simulink library "BrickPi"  (R2018b)
settings: Solver=VariableStepAuto  StartTime=0.0  StopTime=10.0  RelTol=1e-3
libraries: raspberrypilib x50, hdlsllib x27, xpcutilitieslib x18, $bdroot x1
(part 1 of 4)
settings Model: Creator=Isshu  LastModifiedBy=Isshu

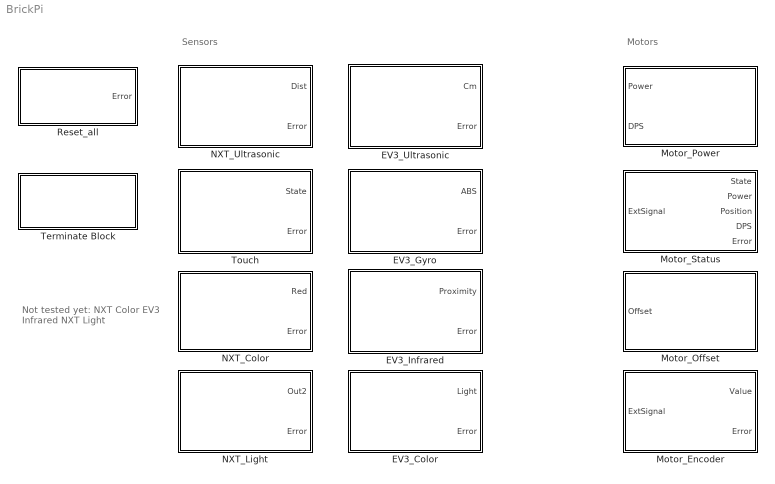
== system BrickPi ==
  note: Not tested yet:
      |
      | NXT Color
      | EV3 Infrared
      | NXT Light
  note: Sensors
  note: Motors
  EV3_Color : Subsystem  mask{SensorPort=1, SensorType=SENSOR_TYPE_EV3_COLOR_AMBIENT}
      mask prompts: SensorPort "Sensor Port"; SensorType "Sensor Type"
      mask init:
      | switch SensorType
      |     case 1, 2
      |         replace_block([gcb, '/Light'],'Terminator','Outport','noprompt')
      |         replace_block([gcb, '/Color_val'],'Outport','Terminator','noprompt')
      |         replace_block([gcb, '/Raw_red'],'Outport','Terminator','noprompt')
      |         replace_block([gcb, '/Red'],'Outport','Terminator','noprompt')
      |         replace_block([gcb, '/Green'],'Outport','Terminator','noprompt')
      |         replace_block([gcb, '/Blue'],'Outport','Terminator','noprompt')
      |         
      |         set_param([gcb, '/Light'],'Port','1')
      |         set_param([gcb, '/Error'],'Port','2')
      |     case 3
      |         replace_block([gcb, '/Light'],'Outport','Terminator','noprompt')
      |         replace_block([gcb, '/Color_val'],'Terminator','Outport','noprompt')
      |         replace_block([gcb, '/Raw_red'],'Outport','Terminator','noprompt')
      |         replace_block([gcb, '/Red'],'Outport','Terminator','noprompt')
      |         replace_block([gcb, '/Green'],'Outport','Terminator','noprompt')
      |         replace_block([gcb, '/Blue'],'Outport','Terminator','noprompt')
      |         
      |         set_param([gcb, '/Color_val'],'Port','1')
      |         set_param([gcb, '/Error'],'Port','2')
      |     case 4
      |         replace_block([gcb, '/Light'],'Outport','Terminator','noprompt')
      |         replace_block([gcb, '/Color_val'],'Outport','Terminator','noprompt')
      |         replace_block([gcb, '/Raw_red'],'Terminator','Outport','noprompt')
      |         replace_block([gcb, '/Red'],'Outport','Terminator','noprompt')
      |         replace_block([gcb, '/Green'],'Outport','Terminator','noprompt')
      |         replace_block([gcb, '/Blue'],'Outport','Terminator','noprompt')
      |         
      |         set_param([gcb, '/Raw_red'],'Port','1')
      |         set_param([gcb, '/Error'],'Port','2')
      |     case 5
      |         replace_block([gcb, '/Light'],'Outport','Terminator','noprompt')
      |         replace_block([gcb, '/Color_val'],'Outport','Terminator','noprompt')
      |         replace_block([gcb, '/Raw_red'],'Outport','Terminator','noprompt')
      |         replace_block([gcb, '/Red'],'Terminator','Outport','noprompt')
      |         replace_block([gcb, '/Green'],'Terminator','Outport','noprompt')
      |         replace_block([gcb, '/Blue'],'Terminator','Outport','noprompt')
      |         
      |         set_param([gcb, '/Red'],'Port','1')
      |         set_param([gcb, '/Green'],'Port','2')
      |         set_param([gcb, '/Blue'],'Port','3')
      |         set_param([gcb, '/Error'],'Port','4')
      | end
      mask TypeOptions SensorPort: 1 | 2 | 3 | 4
      mask TypeOptions SensorType: SENSOR_TYPE_EV3_COLOR_REFLECTED | SENSOR_TYPE_EV3_COLOR_AMBIENT | SENSOR_TYPE_EV3_COLOR_COLOR | SENSOR_TYPE_EV3_COLOR_RAW_REFLECTED | SENSOR_TYPE_EV3_COLOR_COLOR_COMPONENTS
      mask DialogControl DescGroupVar Prompt: EV3 Color Sensor
      mask DialogControl DescTextVar Prompt: <p>         <u>         REFLECTED/ AMBIENT:         </u> <br>         Returns 8 bit integer value for relected light/ light.     </p>     <p>         <u>         COLOR:         </u> <br>         Returns 8 bit integer corresponding to following colors:     </p>         <ul>             <li>0 = No Color</li>             <li>1 = Black</li>             <li>2 = Blue</li>             <li>3 = Green</li>             <li>4 = Yellow</li>             <li>5 = Red</li>             <li>6 = White</li>             <li>7 = Brown</li>         </ul>     <p>         <u>         RAW_REFLECTED:         </u> <br>         Returns 16 bit integer value for measured light.     </p>     <p>         <u>         COLOR_COMPONENTS:         </u> <br>         Returns three 16 bit integer values for red, green and blue and measured light.     </p>
      mask Display:
      | msg = 'EV3 Color\nSensor';
      | switch SensorType
      |     case 1
      |         port_label('output',1,'Light');
      |         port_label('output',2,'Error');
      |     case 2
      |         port_label('output',1,'Light');
      |         port_label('output',2,'Error');
      |     case 3
      |         port_label('output',1,'Color_val');
      |         port_label('output',2,'Error');
      |     case 4
      |         port_label('output',1,'Raw_red');
      |         port_label('output',2,'Error');
      |     case 5
      |         port_label('output',1,'Red');
      |         port_label('output',2,'Green');
      |         port_label('output',3,'Blue');
      |         port_label('output',4,'Error');
      | end
      | 
      | switch SensorPort
      |     case 1
      |         msg = [msg, '\n\nPORT 1'];
      |     case 2
      |         msg = [msg, '\n\nPORT 2'];
      |     case 3
      |         msg = [msg, '\n\nPORT 3'];
      |     case 4
      |         msg = [msg, '\n\nPORT 4'];
      | end
      | 
      | disp(msg);
  EV3_Gyro : Subsystem  mask{SensorPort=1, SensorType=SENSOR_TYPE_EV3_GYRO_ABS}
      mask prompts: SensorPort "Sensor Port"; SensorType "Sensor Type"
      mask init:
      | switch SensorType
      |     case 1
      |         replace_block([gcb, '/ABS'],'Terminator','Outport','noprompt')
      |         replace_block([gcb, '/DPS'],'Outport','Terminator','noprompt')
      |         set_param([gcb, '/ABS'],'Port','1')
      |         set_param([gcb, '/Error'],'Port','2')
      |     case 2
      |         replace_block([gcb, '/ABS'],'Outport','Terminator','noprompt')
      |         replace_block([gcb, '/DPS'],'Terminator','Outport','noprompt')
      |         set_param([gcb, '/DPS'],'Port','1')
      |         set_param([gcb, '/Error'],'Port','2')
      |     case 3
      |         replace_block([gcb, '/ABS'],'Terminator','Outport','noprompt')
      |         replace_block([gcb, '/DPS'],'Terminator','Outport','noprompt')
      |         set_param([gcb, '/ABS'],'Port','1')
      |         set_param([gcb, '/DPS'],'Port','2')
      |         set_param([gcb, '/Error'],'Port','3')
      | end
      mask TypeOptions SensorPort: 1 | 2 | 3 | 4
      mask TypeOptions SensorType: SENSOR_TYPE_EV3_GYRO_ABS | SENSOR_TYPE_EV3_GYRO_DPS | SENSOR_TYPE_EV3_GYRO_ABS_DPS
      mask DialogControl DescGroupVar Prompt: EV3 Gyro Sensor
      mask DialogControl DescTextVar Prompt: <p>         <u>         ABS:         </u> <br>         Returns 16 bit integer value for measured gyro angle in deg.     </p>     <p>         <u>         DPS:         </u> <br>         Returns 16 bit integer value for measured gyro angle velocity in deg/s.     </p>     <p>         <u>         ABD_DPS:         </u> <br>         Returns two 16 bit integer values, one for gyro angle and one for gyro angle velocity.     </p>
      mask Display:
      | msg = 'EV3 Gyro\nSensor';
      | switch SensorType
      |     case 1
      |         port_label('output',1,'ABS');
      |         port_label('output',2,'Error');
      |     case 2
      |         port_label('output',1,'DPS');
      |         port_label('output',2,'Error');
      |     case 3
      |         port_label('output',1,'ABS');
      |         port_label('output',2,'DPS');
      |         port_label('output',3,'Error');
      | end
      | 
      | switch SensorPort
      |     case 1
      |         msg = [msg, '\n\nPORT 1'];
      |     case 2
      |         msg = [msg, '\n\nPORT 2'];
      |     case 3
      |         msg = [msg, '\n\nPORT 3'];
      |     case 4
      |         msg = [msg, '\n\nPORT 4'];
      | end
      | 
      | disp(msg);
  EV3_Infrared : Subsystem  mask{SensorPort=1, SensorType=SENSOR_TYPE_EV3_INFRARED_PROXIMITY}
      mask prompts: SensorPort "Sensor Port"; SensorType "Sensor Type"
      mask init:
      | switch SensorType
      |     case 1
      |         replace_block([gcb, '/Proximity'],'Terminator','Outport','noprompt')
      |         replace_block([gcb, '/Heading'],'Outport','Terminator','noprompt')
      |         replace_block([gcb, '/Distance'],'Outport','Terminator','noprompt')
      |         replace_block([gcb, '/Remote'],'Outport','Terminator','noprompt')
      |         set_param([gcb, '/Proximity'],'Port','1')
      |         set_param([gcb, '/Error'],'Port','2')
      |     case 2
      |         replace_block([gcb, '/Proximity'],'Outport','Terminator','noprompt')
      |         replace_block([gcb, '/Heading'],'Terminator','Outport','noprompt')
      |         replace_block([gcb, '/Distance'],'Terminator','Outport','noprompt')
      |         replace_block([gcb, '/Remote'],'Outport','Terminator','noprompt')
      |         set_param([gcb, '/Heading'],'Port','1')
      |         set_param([gcb, '/Distance'],'Port','2')
      |         set_param([gcb, '/Error'],'Port','3')
      |     case 3
      |         replace_block([gcb, '/Proximity'],'Outport','Terminator','noprompt')
      |         replace_block([gcb, '/Heading'],'Outport','Terminator','noprompt')
      |         replace_block([gcb, '/Distance'],'Outport','Terminator','noprompt')
      |         replace_block([gcb, '/Remote'],'Terminator','Outport','noprompt')
      |         set_param([gcb, '/Remote'],'Port','1')
      |         set_param([gcb, '/Error'],'Port','2')
      | end
      mask TypeOptions SensorPort: 1 | 2 | 3 | 4
      mask TypeOptions SensorType: SENSOR_TYPE_EV3_INFRARED_PROXIMITY | SENSOR_TYPE_EV3_INFRARED_SEEK | SENSOR_TYPE_EV3_INFRARED_REMOTE
      mask Display:
      | msg = 'EV3 Infrared\nSensor';
      | switch SensorType
      |     case 1
      |         port_label('output',1,'Proximity');
      |         port_label('output',2,'Error');
      |     case 2
      |         port_label('output',1,'Heading');
      |         port_label('output',2,'Distance');
      |         port_label('output',3,'Error');
      |     case 3
      |         port_label('output',1,'Remote');
      |         port_label('output',2,'Error');
      | end
      | 
      | switch SensorPort
      |     case 1
      |         msg = [msg, '\n\nPORT 1'];
      |     case 2
      |         msg = [msg, '\n\nPORT 2'];
      |     case 3
      |         msg = [msg, '\n\nPORT 3'];
      |     case 4
      |         msg = [msg, '\n\nPORT 4'];
      | end
      | 
      | disp(msg);
  EV3_Ultrasonic : Subsystem  mask{SensorPort=1, SensorType=SENSOR_TYPE_EV3_ULTRASONIC_CM}
      mask prompts: SensorPort "Sensor Port"; SensorType "Sensor Type"
      mask init:
      | switch SensorType
      |     case 1
      |         replace_block([gcb, '/Cm'],'Terminator','Outport','noprompt')
      |         replace_block([gcb, '/Inches'],'Outport','Terminator','noprompt')
      |         replace_block([gcb, '/Pres'],'Outport','Terminator','noprompt')
      |         set_param([gcb, '/Cm'],'Port','1')
      |         set_param([gcb, '/Error'],'Port','2')
      |     case 2
      |         replace_block([gcb, '/Cm'],'Outport','Terminator','noprompt')
      |         replace_block([gcb, '/Inches'],'Terminator','Outport','noprompt')
      |         replace_block([gcb, '/Pres'],'Outport','Terminator','noprompt')
      |         set_param([gcb, '/Inches'],'Port','1')
      |         set_param([gcb, '/Error'],'Port','2')
      |     case 3
      |         replace_block([gcb, '/Cm'],'Outport','Terminator','noprompt')
      |         replace_block([gcb, '/Inches'],'Outport','Terminator','noprompt')
      |         replace_block([gcb, '/Pres'],'Terminator','Outport','noprompt')
      |         set_param([gcb, '/Pres'],'Port','1')
      |         set_param([gcb, '/Error'],'Port','2')
      | end
      mask TypeOptions SensorPort: 1 | 2 | 3 | 4
      mask TypeOptions SensorType: SENSOR_TYPE_EV3_ULTRASONIC_CM | SENSOR_TYPE_ EV3_ULTRASONIC_INCHES | SENSOR_TYPE_EV3_ULTRASONIC_LISTEN
      mask DialogControl DescGroupVar Prompt: EV3 Ultrasonic Sensor
      mask DialogControl DescTextVar Prompt: <p>         <u>         CM/ INCHES:         </u> <br>         Returns 16 bit float value for measured distance in cm/ inches.     </p>     <p>         <u>         LISTEN:         </u> <br>         Returns boolean value for presence.     </p>
      mask Display:
      | msg = 'EV3 Ultrasonic\nSensor';
      | 
      | switch SensorType
      |     case 1
      |         port_label('output',1,'Cm');
      |         port_label('output',2,'Error');
      |     case 2
      |         port_label('output',1,'Inches');
      |         port_label('output',2,'Error');
      |     case 3
      |         port_label('output',1,'Pres');
      |         port_label('output',2,'Error');
      | end
      | 
      | switch SensorPort
      |     case 1
      |         msg = [msg, '\n\nPORT 1'];
      |     case 2
      |         msg = [msg, '\n\nPORT 2'];
      |     case 3
      |         msg = [msg, '\n\nPORT 3'];
      |     case 4
      |         msg = [msg, '\n\nPORT 4'];
      | end
      | 
      | disp(msg);
  Motor_Encoder : Subsystem  mask{MotorPort=A, ResetMode=Reset on external signal}
      mask prompts: MotorPort "Motor Port"; ResetMode "Encoder Reset"
      mask init:
      | switch ResetMode
      |     case 1
      |         replace_block([gcb,'/ExtSignal'],'Ground','Inport','noprompt')
      |     otherwise
      |         replace_block([gcb,'/ExtSignal'],'Inport','Ground','noprompt')
      | end
      mask TypeOptions MotorPort: A | B | C | D
      mask TypeOptions ResetMode: Reset on external signal | Never reset
      mask DialogControl DescGroupVar Prompt: Get Motor Encoder
      mask DialogControl DescTextVar Prompt: <p>         Optionally one can decide whether the motor encoder is reset while program is running. For example use "Pulse generator" to reset encoder every fixed timestep.     </p>          <p>         Returns int32 value for motor encoder value.     </p>
      mask Display:
      | msg = 'Get Motor\nEncoder';
      | port_label('output',1,'Value');
      | port_label('output',2,'Error');
      | 
      | if ResetMode==1
      |         port_label('input',1,'Reset');
      | end
      | 
      | switch MotorPort
      |     case 1
      |         msg = [msg, '\n\nPORT A'];
      |     case 2
      |         msg = [msg, '\n\nPORT B'];
      |     case 3
      |         msg = [msg, '\n\nPORT C'];
      |     case 4
      |         msg = [msg, '\n\nPORT D'];
      | end
      | 
      | disp(msg);
  Motor_Offset : Subsystem  mask{MotorPort=A}
      mask prompts: MotorPort "Motor Port"
      mask TypeOptions MotorPort: A | B | C | D
      mask DialogControl DescGroupVar Prompt: Set Motor Offset
      mask DialogControl DescTextVar Prompt: <p>         Set int32 value for motor encoder offset.     </p>
      mask Display:
      | port_label('input',1,'Offset');
      | msg = 'Set Motor\nOffset';
      | 
      | switch MotorPort
      |     case 1
      |         msg = [msg, '\n\nPORT A'];
      |     case 2
      |         msg = [msg, '\n\nPORT B'];
      |     case 3
      |         msg = [msg, '\n\nPORT C'];
      |     case 4
      |         msg = [msg, '\n\nPORT D'];
      | end
      | 
      | disp(msg);
  Motor_Power : Subsystem  mask{MotorPort=A, choice=Limits, Kp=0, Kd=0, Kp_DPS=0, Kd_DPS=0}
      mask prompts: MotorPort "Motor Port"; choice "Set Motor"; Kp_DPS "Kp for DPS"; Kd_DPS "Kp for DPS"
      mask init:
      | switch choice
      |     case 1
      |         replace_block([gcb, '/Power'],'Ground','Inport','noprompt')
      |         replace_block([gcb, '/Position'],'Inport','Ground','noprompt')
      |         replace_block([gcb, '/DPS'],'Inport','Ground','noprompt')
      |         
      |         set_param([gcb, '/Power'],'Port','1')
      |     case 2
      |         replace_block([gcb, '/Power'],'Inport','Ground','noprompt')
      |         replace_block([gcb, '/Position'],'Ground','Inport','noprompt')
      |         replace_block([gcb, '/DPS'],'Inport','Ground','noprompt')
      |         
      |         set_param([gcb, '/Position'],'Port','1')
      |     case 3
      |         replace_block([gcb, '/Power'],'Inport','Ground','noprompt')
      |         replace_block([gcb, '/Position'],'Inport','Ground','noprompt')
      |         replace_block([gcb, '/DPS'],'Ground','Inport','noprompt')
      |         
      |         set_param([gcb, '/DPS'],'Port','1')
      |     case 4
      |         replace_block([gcb, '/Power'],'Ground','Inport','noprompt')
      |         replace_block([gcb, '/Position'],'Inport','Ground','noprompt')
      |         replace_block([gcb, '/DPS'],'Ground','Inport','noprompt')
      |         
      |         set_param([gcb, '/Power'],'Port','1')
      |         set_param([gcb, '/DPS'],'Port','2')
      | end
      mask TypeOptions MotorPort: A | B | C | D
      mask TypeOptions choice: Power | Position | DPS | Limits
      mask DialogControl DescGroupVar Prompt: Set Motor Properties
      mask DialogControl DescTextVar Prompt: <p>         <u>POWER</u> <br>         Set 8 bit signed integer value for motor power. -128 stops motor.     </p>     <p>         <u>POSITION</u> <br>         Set 32 bit signed integer value for motor position.     </p>     <p>         <u>DPS</u> <br>         Set 16 bit signed integer value for motor angle velocity.     </p>     <p>         <u>LIMITS</u> <br>         Set 8 bit unsigned integer value for power and 16 bit unsigned integer value for motor angle velocity.     </p> <p>Optionally Kp and Kd values for motor position and dps control can be set. They are set as soon as the values are changed. If every K value is set to zero position control won't work anymore. In that case tune Kp for example to 10. Default values are unfortunately not known.</p>
      mask Display:
      | switch choice
      |     case 1
      |         port_label('input',1,'Power');
      |         msg = 'Set Motor\nPower';
      |     case 2
      |         port_label('input',1,'Position');
      |         msg = 'Set Motor\nPosition';
      |     case 3
      |         port_label('input',1,'DPS');
      |         msg = 'Set Motor\nDPS';
      |     case 4
      |         port_label('input',1,'Power');
      |         port_label('input',2,'DPS');
      |         msg = 'Set Motor\nLimits';
      | end
      | 
      | switch MotorPort
      |     case 1
      |         msg = [msg, '\n\nPORT A'];
      |     case 2
      |         msg = [msg, '\n\nPORT B'];
      |     case 3
      |         msg = [msg, '\n\nPORT C'];
      |     case 4
      |         msg = [msg, '\n\nPORT D'];
      | end
      | 
      | disp(msg);
  Motor_Status : Subsystem  mask{MotorPort=A, ResetMode=Reset on external signal}
      mask prompts: MotorPort "Motor Port"; ResetMode "Encoder Reset"
      mask init:
      | switch ResetMode
      |     case 1
      |         replace_block([gcb,'/ExtSignal'],'Ground','Inport','noprompt')
      |     otherwise
      |         replace_block([gcb,'/ExtSignal'],'Inport','Ground','noprompt')
      | end
      mask TypeOptions MotorPort: A | B | C | D
      mask TypeOptions ResetMode: Reset on external signal | Never reset
      mask DialogControl DescGroupVar Prompt: Get Motor Status
      mask DialogControl DescTextVar Prompt: <p>         Returns uint8 integer value for motor state, int8 value for power, int32 value for position and int16 value for motor angle velocity.     </p>          <p>         Optionally one can decide whether the motor encoder is reset while program is running. For example use "Pulse generator" to reset encoder every fixed timestep.     </p>
      mask Display:
      | msg = 'Get Motor\nStatus';
      | port_label('output',1,'State');
      | port_label('output',2,'Power');
      | port_label('output',3,'Position');
      | port_label('output',4,'DPS');
      | port_label('output',5,'Error');
      | 
      | if ResetMode==1
      |         port_label('input',1,'Reset');
      | end
      | 
      | switch MotorPort
      |     case 1
      |         msg = [msg, '\n\nPORT A'];
      |     case 2
      |         msg = [msg, '\n\nPORT B'];
      |     case 3
      |         msg = [msg, '\n\nPORT C'];
      |     case 4
      |         msg = [msg, '\n\nPORT D'];
      | end
      | 
      | disp(msg);
  NXT_Color : Subsystem  mask{SensorPort=1, SensorType=SENSOR_TYPE_NXT_COLOR_RED}
      mask prompts: SensorPort "Sensor Port"; SensorType "Sensor Type"
      mask init:
      | switch SensorType
      |     case 1
      |         replace_block([gcb, '/Red'],'Terminator','Outport','noprompt')
      |         replace_block([gcb, '/Green'],'Outport','Terminator','noprompt')
      |         replace_block([gcb, '/Blue'],'Outport','Terminator','noprompt')
      |         replace_block([gcb, '/Color'],'Outport','Terminator','noprompt')
      |         replace_block([gcb, '/Ambient'],'Outport','Terminator','noprompt')
      |         
      |         set_param([gcb, '/Red'],'Port','1')
      |         set_param([gcb, '/Error'],'Port','2')
      |     case 2
      |         replace_block([gcb, '/Red'],'Outport','Terminator','noprompt')
      |         replace_block([gcb, '/Green'],'Terminator','Outport','noprompt')
      |         replace_block([gcb, '/Blue'],'Outport','Terminator','noprompt')
      |         replace_block([gcb, '/Color'],'Outport','Terminator','noprompt')
      |         replace_block([gcb, '/Ambient'],'Outport','Terminator','noprompt')
      |         
      |         set_param([gcb, '/Green'],'Port','1')
      |         set_param([gcb, '/Error'],'Port','2')
      |     case 3
      |         replace_block([gcb, '/Red'],'Outport','Terminator','noprompt')
      |         replace_block([gcb, '/Green'],'Outport','Terminator','noprompt')
      |         replace_block([gcb, '/Blue'],'Terminator','Outport','noprompt')
      |         replace_block([gcb, '/Color'],'Outport','Terminator','noprompt')
      |         replace_block([gcb, '/Ambient'],'Outport','Terminator','noprompt')
      |         
      |         set_param([gcb, '/Blue'],'Port','1')
      |         set_param([gcb, '/Error'],'Port','2')
      |     case 4
      |         replace_block([gcb, '/Red'],'Terminator','Outport','noprompt')
      |         replace_block([gcb, '/Green'],'Terminator','Outport','noprompt')
      |         replace_block([gcb, '/Blue'],'Terminator','Outport','noprompt')
      |         replace_block([gcb, '/Color'],'Terminator','Outport','noprompt')
      |         replace_block([gcb, '/Ambient'],'Terminator','Outport','noprompt')
      |         
      |         set_param([gcb, '/Red'],'Port','1')
      |         set_param([gcb, '/Green'],'Port','2')
      |         set_param([gcb, '/Blue'],'Port','3')
      |         set_param([gcb, '/Color'],'Port','4')
      |         set_param([gcb, '/Ambient'],'Port','5')
      |         set_param([gcb, '/Error'],'Port','6')
      |     case 5
      |         replace_block([gcb, '/Red'],'Outport','Terminator','noprompt')
      |         replace_block([gcb, '/Green'],'Outport','Terminator','noprompt')
      |         replace_block([gcb, '/Blue'],'Outport','Terminator','noprompt')
      |         replace_block([gcb, '/Color'],'Outport','Terminator','noprompt')
      |         replace_block([gcb, '/Ambient'],'Terminator','Outport','noprompt')
      |         
      |         set_param([gcb, '/Ambient'],'Port','1')
      |         set_param([gcb, '/Error'],'Port','2')
      | end
      mask TypeOptions SensorPort: 1 | 2 | 3 | 4
      mask TypeOptions SensorType: SENSOR_TYPE_NXT_COLOR_RED | SENSOR_TYPE_NXT_COLOR_GREEN | SENSOR_TYPE_NXT_COLOR_BLUE | SENSOR_TYPE_NXT_COLOR_FULL | SENSOR_TYPE_NXT_COLOR_OFF
      mask DialogControl DescGroupVar Prompt: NXT Color Sensor
      mask DialogControl DescTextVar Prompt: <p>         <u>         RED/ GREEN/ BLUE/ OFF:         </u> <br>         Returns 16 bit integer value for red/ green/ blue/ measured light.     </p>     <p>         <u>         FULL:         </u> <br>         Returns one 8 bit value for color corresponding to following colors and four 16 bit integer values for red, green, blue and measured light.     </p>     <ul>             <li>0 = No Color</li>             <li>1 = Black</li>             <li>2 = Blue</li>             <li>3 = Green</li>             <li>4 = Yellow</li>             <li>5 = Red</li>             <li>6 = White</li>             <li>7 = Brown</li>     </ul>
      mask Display:
      | msg = 'NXT Color\nSensor';
      | switch SensorType
      |     case 1
      |         port_label('output',1,'Red');
      |         port_label('output',2,'Error');
      |     case 2
      |         port_label('output',1,'Green');
      |         port_label('output',2,'Error');
      |     case 3
      |         port_label('output',1,'Blue');
      |         port_label('output',2,'Error');
      |     case 4
      |         port_label('output',1,'Red');
      |         port_label('output',2,'Green');
      |         port_label('output',3,'Blue');
      |         port_label('output',4,'Color');
      |         port_label('output',5,'Ambient');
      |         port_label('output',6,'Error');
      |     case 5
      |         port_label('output',1,'Amb');
      |         port_label('output',2,'Error');
      | end
      | 
      | switch SensorPort
      |     case 1
      |         msg = [msg, '\n\nPORT 1'];
      |     case 2
      |         msg = [msg, '\n\nPORT 2'];
      |     case 3
      |         msg = [msg, '\n\nPORT 3'];
      |     case 4
      |         msg = [msg, '\n\nPORT 4'];
      | end
      | 
      | disp(msg);
  NXT_Light : Subsystem  mask{SensorPort=1, SensorType=SENSOR_TYPE_NXT_LIGHT_ON}
      mask prompts: SensorPort "Sensor Port"; SensorType "Sensor Type"
      mask TypeOptions SensorPort: 1 | 2 | 3 | 4
      mask TypeOptions SensorType: SENSOR_TYPE_NXT_LIGHT_ON | SENSOR_TYPE_NXT_LIGHT_OFF
      mask DialogControl DescGroupVar Prompt: NXT Light Sensor
      mask DialogControl DescTextVar Prompt: <p>         <u>         ON/ OFF:         </u> <br>         Returns 16 bit integer value for reflected/ measured light.     </p>
      mask Display:
      | msg = 'NXT Light\nSensor';
      | port_label('output',1,'Light');
      | port_label('output',2,'Error');
      | 
      | switch SensorPort
      |     case 1
      |         msg = [msg, '\n\nPORT 1'];
      |     case 2
      |         msg = [msg, '\n\nPORT 2'];
      |     case 3
      |         msg = [msg, '\n\nPORT 3'];
      |     case 4
      |         msg = [msg, '\n\nPORT 4'];
      | end
      | 
      | disp(msg);
  NXT_Ultrasonic : Subsystem  mask{SensorPort=1}
      mask prompts: SensorPort "Sensor Port"
      mask TypeOptions SensorPort: 1 | 2 | 3 | 4
      mask DialogControl DescGroupVar Prompt: NXT Ultrasonic Sensor
      mask DialogControl DescTextVar Prompt: <p>     Returns measured distance in cm as a 8 bit integer value. </p>
      mask Display:
      | msg = 'NXT Ultrasonic\nSensor';
      | port_label('output',1,'Dist');
      | port_label('output',2,'Error');
      | 
      | switch SensorPort
      |     case 1
      |         msg = [msg, '\n\nPORT 1'];
      |     case 2
      |         msg = [msg, '\n\nPORT 2'];
      |     case 3
      |         msg = [msg, '\n\nPORT 3'];
      |     case 4
      |         msg = [msg, '\n\nPORT 4'];
      | end
      | 
      | disp(msg);
  Reset_all : Subsystem
      mask DialogControl DescGroupVar Prompt: Reset
      mask DialogControl DescTextVar Prompt: Sets motor power to -128 (no motion) and resets sensor types assigned to ports
      mask Display: disp('Reset all')
  Terminate Block : Subsystem  TreatAsAtomicUnit=on
  Touch : Subsystem  mask{SensorPort=1, SensorType=SENSOR_TYPE_TOUCH_NXT}
      mask prompts: SensorPort "Sensor Port"; SensorType "Sensor Type"
      mask TypeOptions SensorPort: 1 | 2 | 3 | 4
      mask TypeOptions SensorType: SENSOR_TYPE_TOUCH_NXT | SENSOR_TYPE_TOUCH_EV3
      mask DialogControl DescGroupVar Prompt: NXT/EV3 Touch Sensor
      mask DialogControl DescTextVar Prompt: <p>     Doesn't work if the wrong sensor type (NXT or EV3) is selected. </p> <p>     Returns boolean value for button pushed (1) or not (0). </p>
      mask Display:
      | msg = 'NXT/ EV3 Touch\nSensor';
      | port_label('output',1,'State');
      | port_label('output',2,'Error');
      | 
      | switch SensorPort
      |     case 1
      |         msg = [msg, '\n\nPORT 1'];
      |     case 2
      |         msg = [msg, '\n\nPORT 2'];
      |     case 3
      |         msg = [msg, '\n\nPORT 3'];
      |     case 4
      |         msg = [msg, '\n\nPORT 4'];
      | end
      | 
      | disp(msg);

== system BrickPi/EV3_Color ==
  AND : Logic  AllPortsSameDT=off  OutDataTypeStr=boolean
  Blue : Terminator
  Color_val : Terminator
  Constant : Constant
  Demux : Demux  Outputs=3
  Get_sensor_value : Subsystem
  Green : Terminator
  Memory : Memory
  Mux : Mux  Inputs=2
  NOT : Logic  Operator=NOT  IconShape=distinctive  AllPortsSameDT=off  OutDataTypeStr=boolean
  NOT1 : Logic  Operator=NOT  IconShape=distinctive  AllPortsSameDT=off  OutDataTypeStr=boolean
  Raw_red : Terminator
  Red : Terminator
  SensorPort : Constant  Value=SensorPort  OutDataTypeStr=uint8
  SensorType : Constant  Value=SensorType  OutDataTypeStr=uint8
  Set_sensor_type : Subsystem  Priority=21
  Light : Outport
  Error : Outport  Port=2
  wires:
  SensorType/1 -> Get_sensor_value/2(SensorType), Set_sensor_type/2(SensorType)
  NOT/1 -> Set_sensor_type/Enable
  Mux/1 -> Error/1
  Constant/1 -> Memory/1
  Get_sensor_value/5(Error) -> Mux/2
  Memory/1 -> NOT/1, AND/2
  AND/1 -> Get_sensor_value/Enable
  SensorPort/1 -> Set_sensor_type/1(SensorPort), Get_sensor_value/1(SensorPort)
  Get_sensor_value/1(Light) -> Light/1
  Set_sensor_type/1(Error) -> NOT1/1, Mux/1
  NOT1/1 -> AND/1
  Demux/1 -> Red/1
  Demux/2 -> Green/1
  Demux/3 -> Blue/1
  Get_sensor_value/4(Color) -> Demux/1
  Get_sensor_value/2(Color_val) -> Color_val/1
  Get_sensor_value/3(Raw_red) -> Raw_red/1

== system BrickPi/EV3_Gyro ==
  AND : Logic  AllPortsSameDT=off  OutDataTypeStr=boolean
  Constant : Constant
  DPS : Terminator
  Get_sensor_value : Subsystem
  Memory : Memory
  Mux : Mux  Inputs=2
  NOT : Logic  Operator=NOT  IconShape=distinctive  AllPortsSameDT=off  OutDataTypeStr=boolean
  NOT1 : Logic  Operator=NOT  IconShape=distinctive  AllPortsSameDT=off  OutDataTypeStr=boolean
  SensorPort : Constant  Value=SensorPort  OutDataTypeStr=uint8
  SensorType : Constant  Value=SensorType  OutDataTypeStr=uint8
  Set_sensor_type : Subsystem  Priority=21
  ABS : Outport
  Error : Outport  Port=2
  wires:
  SensorType/1 -> Get_sensor_value/2(SensorType), Set_sensor_type/2(SensorType)
  NOT/1 -> Set_sensor_type/Enable
  Mux/1 -> Error/1
  Constant/1 -> Memory/1
  Get_sensor_value/3(Error) -> Mux/2
  Memory/1 -> NOT/1, AND/2
  AND/1 -> Get_sensor_value/Enable
  SensorPort/1 -> Set_sensor_type/1(SensorPort), Get_sensor_value/1(SensorPort)
  Set_sensor_type/1(Error) -> NOT1/1, Mux/1
  NOT1/1 -> AND/1
  Get_sensor_value/1(ABS) -> ABS/1
  Get_sensor_value/2(DPS) -> DPS/1

== system BrickPi/EV3_Infrared ==
  AND : Logic  AllPortsSameDT=off  OutDataTypeStr=boolean
  Constant : Constant
  Distance : Terminator
  Get_sensor_value : Subsystem
  Heading : Terminator
  Memory : Memory
  Mux : Mux  Inputs=2
  NOT : Logic  Operator=NOT  IconShape=distinctive  AllPortsSameDT=off  OutDataTypeStr=boolean
  NOT1 : Logic  Operator=NOT  IconShape=distinctive  AllPortsSameDT=off  OutDataTypeStr=boolean
  Remote : Terminator
  SensorPort : Constant  Value=SensorPort  OutDataTypeStr=uint8
  SensorType : Constant  Value=SensorType  OutDataTypeStr=uint8
  Set_sensor_type : Subsystem  Priority=21
  Proximity : Outport
  Error : Outport  Port=2
  wires:
  Get_sensor_value/1(Proximity) -> Proximity/1
  Mux/1 -> Error/1
  Set_sensor_type/1(Error) -> Mux/1, NOT1/1
  AND/1 -> Get_sensor_value/Enable
  NOT1/1 -> AND/1
  SensorPort/1 -> Get_sensor_value/1(SensorPort), Set_sensor_type/1(SensorPort)
  Memory/1 -> AND/2, NOT/1
  Constant/1 -> Memory/1
  NOT/1 -> Set_sensor_type/Enable
  SensorType/1 -> Set_sensor_type/2(SensorType), Get_sensor_value/2(SensorType)
  Get_sensor_value/5(Error) -> Mux/2
  Get_sensor_value/4(Remote) -> Remote/1
  Get_sensor_value/3(Distance) -> Distance/1
  Get_sensor_value/2(Heading) -> Heading/1

== system BrickPi/EV3_Ultrasonic ==
  AND : Logic  AllPortsSameDT=off  OutDataTypeStr=boolean
  Constant : Constant
  Get_sensor_value : Subsystem
  Inches : Terminator
  Memory : Memory
  Mux : Mux  Inputs=2
  NOT : Logic  Operator=NOT  IconShape=distinctive  AllPortsSameDT=off  OutDataTypeStr=boolean
  NOT1 : Logic  Operator=NOT  IconShape=distinctive  AllPortsSameDT=off  OutDataTypeStr=boolean
  Pres : Terminator
  SensorPort : Constant  Value=SensorPort  OutDataTypeStr=uint8
  SensorType : Constant  Value=SensorType  OutDataTypeStr=uint8
  Set_sensor_type : Subsystem  Priority=21
  Cm : Outport
  Error : Outport  Port=2
  wires:
  Mux/1 -> Error/1
  Memory/1 -> NOT/1, AND/2
  NOT1/1 -> AND/1
  Get_sensor_value/1(cm) -> Cm/1
  AND/1 -> Get_sensor_value/Enable
  NOT/1 -> Set_sensor_type/Enable
  Get_sensor_value/4(Error) -> Mux/2
  Set_sensor_type/1(Error) -> NOT1/1, Mux/1
  Constant/1 -> Memory/1
  Get_sensor_value/3(pres) -> Pres/1
  SensorPort/1 -> Get_sensor_value/1(SensorPort), Set_sensor_type/1(SensorPort)
  SensorType/1 -> Get_sensor_value/2(SensorType), Set_sensor_type/2(SensorType)
  Get_sensor_value/2(inch) -> Inches/1

== system BrickPi/Motor_Encoder ==
  ExtSignal : Inport
  AND : Logic  IconShape=distinctive  AllPortsSameDT=off  OutDataTypeStr=boolean
  Constant : Constant
  Get Encoder Value : Subsystem
  Memory : Memory
  MotorPort : Constant  Value=MotorPort  OutDataTypeStr=uint8
  NOT : Logic  Operator=NOT  IconShape=distinctive  AllPortsSameDT=off  OutDataTypeStr=boolean
  NOT1 : Logic  Operator=NOT  IconShape=distinctive  AllPortsSameDT=off  OutDataTypeStr=boolean
  Reset Encoder once : Subsystem
  ResetMode : Constant  Value=ResetMode
  Value : Outport
  Error : Outport  Port=2
  wires:
  Get Encoder Value/1(Value) -> Value/1
  Get Encoder Value/2(Error) -> Error/1
  Constant/1 -> Memory/1
  Memory/1 -> NOT1/1, AND/1
  MotorPort/1 -> Get Encoder Value/1(MotorPort), Reset Encoder once/1(MotorPort)
  Reset Encoder once/1(Error) -> NOT/1
  AND/1 -> Get Encoder Value/Enable
  NOT/1 -> AND/2
  ResetMode/1 -> Get Encoder Value/2(ResetMode)
  ExtSignal/1 -> Get Encoder Value/3(ExtSignal)
  NOT1/1 -> Reset Encoder once/Enable

== system BrickPi/Motor_Offset ==
  Offset : Inport  OutDataTypeStr=int32
  If : If  NumInputs=2  IfExpression=u1 ~= u2
  If Action Subsystem : Subsystem  TreatAsAtomicUnit=on
  Memory : Memory
  Terminator : Terminator
  wires:
  If/1 -> If Action Subsystem/Action
  If/2 -> Terminator/1
  Memory/1 -> If/1
  Offset/1 -> If Action Subsystem/1(Offset), If/2, Memory/1

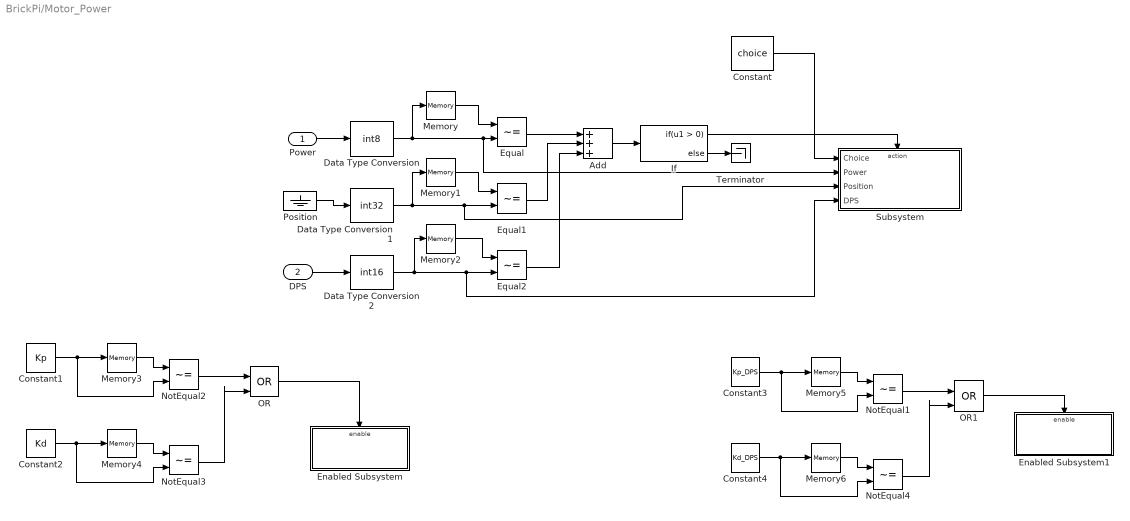
== system BrickPi/Motor_Power ==
  Power : Inport
  DPS : Inport  Port=2
  Add : Sum  Inputs=3
  Constant : Constant  Value=choice
  Constant1 : Constant  Value=Kp
  Constant2 : Constant  Value=Kd
  Constant3 : Constant  Value=Kp_DPS
  Constant4 : Constant  Value=Kd_DPS
  Data Type Conversion : DataTypeConversion  OutDataTypeStr=int8
  Data Type Conversion1 : DataTypeConversion  OutDataTypeStr=int32
  Data Type Conversion2 : DataTypeConversion  OutDataTypeStr=int16
  Enabled Subsystem : Subsystem  TreatAsAtomicUnit=on
  Enabled Subsystem1 : Subsystem  TreatAsAtomicUnit=on
  Equal : RelationalOperator  Operator=~=  RndMeth=Simplest
  Equal1 : RelationalOperator  Operator=~=  RndMeth=Simplest
  Equal2 : RelationalOperator  Operator=~=  RndMeth=Simplest
  If : If
  Memory : Memory  InheritSampleTime=on
  Memory1 : Memory  InheritSampleTime=on
  Memory2 : Memory  InheritSampleTime=on
  Memory{3..6} (4 alike) : Memory
  NotEqual{1..4} (4 alike) : RelationalOperator  Operator=~=  OutDataTypeStr=boolean  RndMeth=Simplest
  OR : Logic  Operator=OR  IconShape=distinctive  AllPortsSameDT=off  OutDataTypeStr=boolean
  OR1 : Logic  Operator=OR  IconShape=distinctive  AllPortsSameDT=off  OutDataTypeStr=boolean
  Position : Ground
  Subsystem : Subsystem
  Terminator : Terminator
  wires:
  Memory6/1 -> NotEqual4/1
  Constant3/1 -> NotEqual1/2, Memory5/1
  Constant4/1 -> Memory6/1, NotEqual4/2
  NotEqual1/1 -> OR1/1
  NotEqual4/1 -> OR1/2
  NotEqual3/1 -> OR/2
  Memory5/1 -> NotEqual1/1
  OR1/1 -> Enabled Subsystem1/Enable
  OR/1 -> Enabled Subsystem/Enable
  Memory3/1 -> NotEqual2/1
  Memory4/1 -> NotEqual3/1
  NotEqual2/1 -> OR/1
  Constant1/1 -> NotEqual2/2, Memory3/1
  Constant2/1 -> Memory4/1, NotEqual3/2
  Equal/1 -> Add/1
  Data Type Conversion1/1 -> Memory1/1, Subsystem/3(Position), Equal1/2
  If/2 -> Terminator/1
  Constant/1 -> Subsystem/1(Choice)
  Memory1/1 -> Equal1/1
  Data Type Conversion2/1 -> Memory2/1, Subsystem/4(DPS), Equal2/2
  Data Type Conversion/1 -> Memory/1, Subsystem/2(Power), Equal/2
  Add/1 -> If/1
  Position/1 -> Data Type Conversion1/1
  Equal1/1 -> Add/2
  Memory2/1 -> Equal2/1
  Equal2/1 -> Add/3
  DPS/1 -> Data Type Conversion2/1
  If/1 -> Subsystem/Action
  Memory/1 -> Equal/1
  Power/1 -> Data Type Conversion/1

== system BrickPi/Motor_Status ==
  ExtSignal : Inport
  AND : Logic  IconShape=distinctive  AllPortsSameDT=off  OutDataTypeStr=boolean
  Constant : Constant
  Get motor values : Subsystem
  Memory : Memory
  MotorPort : Constant  Value=MotorPort  OutDataTypeStr=uint8
  NOT : Logic  Operator=NOT  IconShape=distinctive  AllPortsSameDT=off  OutDataTypeStr=boolean
  NOT1 : Logic  Operator=NOT  IconShape=distinctive  AllPortsSameDT=off  OutDataTypeStr=boolean
  Reset Encoder once : Subsystem
  ResetMode : Constant  Value=ResetMode  OutDataTypeStr=uint8
  State : Outport
  Power : Outport  Port=2
  Position : Outport  Port=3
  DPS : Outport  Port=4
  Error : Outport  Port=5
  wires:
  Get motor values/1(State) -> State/1
  Get motor values/2(Power) -> Power/1
  Get motor values/3(Position) -> Position/1
  Get motor values/4(DPS) -> DPS/1
  Get motor values/5(Error) -> Error/1
  Constant/1 -> Memory/1
  Memory/1 -> NOT1/1, AND/1
  NOT1/1 -> Reset Encoder once/Enable
  NOT/1 -> AND/2
  Reset Encoder once/1(Error) -> NOT/1
  MotorPort/1 -> Get motor values/1(MotorPort), Reset Encoder once/1(MotorPort)
  ResetMode/1 -> Get motor values/2(ResetMode)
  ExtSignal/1 -> Get motor values/3(ExtSignal)
  AND/1 -> Get motor values/Enable

== system BrickPi/NXT_Color ==
  AND : Logic  AllPortsSameDT=off  OutDataTypeStr=boolean
  Ambient : Terminator
  Blue : Terminator
  Color : Terminator
  Constant : Constant
  Data Type Conversion4 : DataTypeConversion  OutDataTypeStr=int8
  Demux : Demux  Outputs=5
  Get_sensor_value : Subsystem
  Green : Terminator
  Memory : Memory
  Mux : Mux  Inputs=2
  NOT : Logic  Operator=NOT  IconShape=distinctive  AllPortsSameDT=off  OutDataTypeStr=boolean
  NOT1 : Logic  Operator=NOT  IconShape=distinctive  AllPortsSameDT=off  OutDataTypeStr=boolean
  SensorPort : Constant  Value=SensorPort  OutDataTypeStr=uint8
  SensorType : Constant  Value=SensorType  OutDataTypeStr=uint8
  Set_sensor_type : Subsystem  Priority=21
  Red : Outport
  Error : Outport  Port=2
  wires:
  SensorType/1 -> Get_sensor_value/2(SensorType), Set_sensor_type/2(SensorType)
  NOT/1 -> Set_sensor_type/Enable
  Mux/1 -> Error/1
  Constant/1 -> Memory/1
  Get_sensor_value/2(Error) -> Mux/2
  Memory/1 -> NOT/1, AND/2
  AND/1 -> Get_sensor_value/Enable
  SensorPort/1 -> Set_sensor_type/1(SensorPort), Get_sensor_value/1(SensorPort)
  Set_sensor_type/1(Error) -> NOT1/1, Mux/1
  NOT1/1 -> AND/1
  Demux/1 -> Data Type Conversion4/1
  Demux/2 -> Red/1
  Demux/3 -> Green/1
  Demux/4 -> Blue/1
  Demux/5 -> Ambient/1
  Get_sensor_value/1(Values) -> Demux/1
  Data Type Conversion4/1 -> Color/1

== system BrickPi/NXT_Light ==
  AND : Logic  AllPortsSameDT=off  OutDataTypeStr=boolean
  Constant : Constant
  Get_sensor_value : Subsystem
  Memory : Memory
  Mux : Mux  Inputs=2
  NOT : Logic  Operator=NOT  IconShape=distinctive  AllPortsSameDT=off  OutDataTypeStr=boolean
  NOT1 : Logic  Operator=NOT  IconShape=distinctive  AllPortsSameDT=off  OutDataTypeStr=boolean
  SensorPort : Constant  Value=SensorPort  OutDataTypeStr=uint8
  SensorType : Constant  Value=SensorType  OutDataTypeStr=uint8
  Set_sensor_type : Subsystem  Priority=21
  Out2 : Outport
  Error : Outport  Port=2
  wires:
  SensorType/1 -> Get_sensor_value/2(SensorType), Set_sensor_type/2(SensorType)
  NOT/1 -> Set_sensor_type/Enable
  Mux/1 -> Error/1
  Constant/1 -> Memory/1
  Get_sensor_value/2(Error) -> Mux/2
  Memory/1 -> NOT/1, AND/2
  AND/1 -> Get_sensor_value/Enable
  SensorPort/1 -> Set_sensor_type/1(SensorPort), Get_sensor_value/1(SensorPort)
  Get_sensor_value/1(Value) -> Out2/1
  Set_sensor_type/1(Error) -> NOT1/1, Mux/1
  NOT1/1 -> AND/1

== system BrickPi/NXT_Ultrasonic ==
  AND : Logic  AllPortsSameDT=off  OutDataTypeStr=boolean
  Constant : Constant
  Get_sensor_value : Subsystem
  Memory : Memory
  Mux : Mux  Inputs=2
  NOT : Logic  Operator=NOT  IconShape=distinctive  AllPortsSameDT=off  OutDataTypeStr=boolean
  NOT1 : Logic  Operator=NOT  IconShape=distinctive  AllPortsSameDT=off  OutDataTypeStr=boolean
  SensorPort : Constant  Value=SensorPort  OutDataTypeStr=uint8
  Set_sensor_type : Subsystem  Priority=21
  Dist : Outport
  Error : Outport  Port=2
  wires:
  Constant/1 -> Memory/1
  NOT/1 -> Set_sensor_type/Enable
  Memory/1 -> AND/2, NOT/1
  SensorPort/1 -> Get_sensor_value/1(SensorPort), Set_sensor_type/1(SensorPort)
  Get_sensor_value/1(Value) -> Dist/1
  AND/1 -> Get_sensor_value/Enable
  Set_sensor_type/1(Error) -> Mux/1, NOT1/1
  NOT1/1 -> AND/1
  Mux/1 -> Error/1
  Get_sensor_value/2(Error) -> Mux/2

== system BrickPi/Reset_all ==
  OR : Logic  Operator=OR  IconShape=distinctive  AllPortsSameDT=off  OutDataTypeStr=boolean
  Reset motor power : Subsystem
  Reset sensor ports : Subsystem
  Error : Outport
  wires:
  OR/1 -> Error/1
  Reset sensor ports/1(Error) -> OR/1
  Reset motor power/1(Error) -> OR/2

== system BrickPi/Terminate Block ==
  note: Executes "Reset all" at the end of program.
  Event Listener : EventListener  DisableCoverage=on  EventType=Terminate  EventName=reset
  Reset_all : $bdroot/Reset_all

== system BrickPi/Touch ==
  AND : Logic  AllPortsSameDT=off  OutDataTypeStr=boolean
  Constant : Constant
  Get_sensor_value : Subsystem
  Memory : Memory
  Mux : Mux  Inputs=2
  NOT : Logic  Operator=NOT  IconShape=distinctive  AllPortsSameDT=off  OutDataTypeStr=boolean
  NOT1 : Logic  Operator=NOT  IconShape=distinctive  AllPortsSameDT=off  OutDataTypeStr=boolean
  SensorPort : Constant  Value=SensorPort  OutDataTypeStr=uint8
  SensorType : Constant  Value=SensorType  OutDataTypeStr=uint8
  Set_sensor_type : Subsystem  Priority=21
  State : Outport
  Error : Outport  Port=2
  wires:
  NOT1/1 -> AND/1
  Set_sensor_type/1(Error) -> Mux/1, NOT1/1
  Get_sensor_value/1(Value) -> State/1
  SensorPort/1 -> Get_sensor_value/1(SensorPort), Set_sensor_type/1(SensorPort)
  AND/1 -> Get_sensor_value/Enable
  Memory/1 -> AND/2, NOT/1
  Get_sensor_value/2(Error) -> Mux/2
  Constant/1 -> Memory/1
  Mux/1 -> Error/1
  NOT/1 -> Set_sensor_type/Enable
  SensorType/1 -> Set_sensor_type/2(SensorType), Get_sensor_value/2(SensorType)

== system BrickPi/EV3_Color/Get_sensor_value ==
  SensorPort : Inport
  SensorType : Inport  Port=2  OutDataTypeStr=uint8
  Enable : EnablePort
  COLOR_COMPONENTS : Subsystem
  COLOR_RAW_REFLECTED : Subsystem
  COLOR_REF_AMB : Subsystem
  Data Type Conversion : DataTypeConversion  OutDataTypeStr=int8
  Data Type Conversion1 : DataTypeConversion  OutDataTypeStr=int8
  Merge : Merge  Inputs=3
  Switch Case : SwitchCase  CaseConditions={[1,2,3],4,5}
  Terminator : Terminator
  Light : Outport
  Color_val : Outport  Port=2
  Raw_red : Outport  Port=3
  Color : Outport  Port=4
  Error : Outport  Port=5
  wires:
  SensorType/1 -> COLOR_REF_AMB/2(SensorType), COLOR_COMPONENTS/2(SensorType), COLOR_RAW_REFLECTED/2(SensorType), Switch Case/1
  Switch Case/1 -> COLOR_REF_AMB/Action
  Merge/1 -> Error/1
  COLOR_REF_AMB/3(Error) -> Merge/1
  Switch Case/3 -> COLOR_COMPONENTS/Action
  Switch Case/2 -> COLOR_RAW_REFLECTED/Action
  SensorPort/1 -> COLOR_COMPONENTS/1(SensorPort), COLOR_RAW_REFLECTED/1(SensorPort), COLOR_REF_AMB/1(SensorPort)
  COLOR_COMPONENTS/2(Error) -> Merge/3
  COLOR_RAW_REFLECTED/2(Error) -> Merge/2
  Data Type Conversion/1 -> Light/1
  Data Type Conversion1/1 -> Color_val/1
  COLOR_REF_AMB/1(Light) -> Data Type Conversion/1
  COLOR_REF_AMB/2(Color_val) -> Data Type Conversion1/1
  COLOR_COMPONENTS/1(Color) -> Color/1
  COLOR_RAW_REFLECTED/1(Raw_red) -> Raw_red/1
  Switch Case/4 -> Terminator/1

== system BrickPi/EV3_Color/Set_sensor_type ==
  note: Set sensor type
  note: Check whether 4th element == 0xA5?
  SensorPort : Inport  OutDataTypeStr=uint8
  SensorType : Inport  Port=2  OutDataTypeStr=uint8
  Enable : EnablePort
  0xA5 : Constant  Value=165
  Address : Constant  VectorParams1D=off  OutDataTypeStr=uint8
  Constant2 : Constant  OutDataTypeStr=uint8
  Constant3 : Constant  OutDataTypeStr=uint8
  Mux1 : Mux
  NAND : Logic  Operator=NAND  IconShape=distinctive  AllPortsSameDT=off  OutDataTypeStr=boolean
  SPI Master Transfer1 : raspberrypilib/SPI Master Transfer  Priority=1  BoardProperty=Pi 3 Model B  SPIModule=uint32(0)  Mode=Master  BusSpeed=1000000  Pin=SPI0_CE1  FirstBitToTransfer=Most significant bit (MSB)  ClockMode=0  BlockFunction=Transfer  RegisterAddress=0  OutputDataType=int8  OutputDataLength=1
      settings: SourceProductName=Simulink Support Package for Raspberry Pi Hardware  SourceProductBaseCode=RASPPI
  SPI_MSG_SET_ SENSOR_TYPE : Constant  Value=12  OutMin=[1]  OutMax=[28]  OutDataTypeStr=uint8
  Selector1 : Selector  InputPortWidth=4  IndexOptions=Index vector (dialog)  Indices=[4]  OutputSizes=1
  Sensor type offset : Constant  Value=17  OutDataTypeStr=uint8
  Shift Arithmetic : ArithShift  BitShiftNumberSource=Input port  BitShiftNumber=8  BitShiftDirection=Left
      settings: InputPortMap=u0,p1
  Subtract : Sum  Inputs=+-
  Sum : Sum
  Error : Outport  InitialOutput=[1]
  wires:
  Sensor type offset/1 -> Sum/2
  SensorType/1 -> Sum/1
  Sum/1 -> Mux1/4
  Shift Arithmetic/1 -> Mux1/3
  Constant2/1 -> Shift Arithmetic/1
  SensorPort/1 -> Subtract/1
  Constant3/1 -> Subtract/2
  Subtract/1 -> Shift Arithmetic/2
  NAND/1 -> Error/1
  0xA5/1 -> NAND/2
  Selector1/1 -> NAND/1
  SPI_MSG_SET_ SENSOR_TYPE/1 -> Mux1/2
  Address/1 -> Mux1/1
  SPI Master Transfer1/1 -> Selector1/1
  Mux1/1 -> SPI Master Transfer1/1

== system BrickPi/EV3_Gyro/Get_sensor_value ==
  note: Which sensor type has been selected?
  SensorPort : Inport
  SensorType : Inport  Port=2  OutDataTypeStr=uint8
  Enable : EnablePort  StatesWhenEnabling=reset  PropagateVarSize=During execution
  ABS_and_DPS : Subsystem
  ABS_or_DPS : Subsystem
  Merge1 : Merge
  Merge2 : Merge
  Merge3 : Merge
  Switch Case : SwitchCase  CaseConditions={[1,2],3}
  Terminator : Terminator
  ABS : Outport
  DPS : Outport  Port=2
  Error : Outport  Port=3
  wires:
  Switch Case/1 -> ABS_or_DPS/Action
  Switch Case/2 -> ABS_and_DPS/Action
  SensorType/1 -> ABS_and_DPS/2(SensorType), ABS_or_DPS/2(SensorType), Switch Case/1
  Merge2/1 -> ABS/1
  Merge1/1 -> Error/1
  SensorPort/1 -> ABS_and_DPS/1(SensorPort), ABS_or_DPS/1(SensorPort)
  ABS_or_DPS/3(Error) -> Merge1/1
  ABS_and_DPS/3(Error) -> Merge1/2
  Merge3/1 -> DPS/1
  ABS_or_DPS/1(ABS) -> Merge2/1
  ABS_and_DPS/1(ABS) -> Merge2/2
  ABS_and_DPS/2(DPS) -> Merge3/2
  ABS_or_DPS/2(DPS) -> Merge3/1
  Switch Case/3 -> Terminator/1

== system BrickPi/EV3_Gyro/Set_sensor_type ==
  note: Set sensor type
  note: Check whether 4th element == 0xA5?
  SensorPort : Inport  OutDataTypeStr=uint8
  SensorType : Inport  Port=2  OutDataTypeStr=uint8
  Enable : EnablePort  PropagateVarSize=During execution
  0xA5 : Constant  Value=165
  Address : Constant  VectorParams1D=off  OutDataTypeStr=uint8
  Constant2 : Constant  OutDataTypeStr=uint8
  Constant3 : Constant  OutDataTypeStr=uint8
  Mux1 : Mux
  NAND : Logic  Operator=NAND  IconShape=distinctive  AllPortsSameDT=off  OutDataTypeStr=boolean
  SPI Master Transfer1 : raspberrypilib/SPI Master Transfer  Priority=1  BoardProperty=Pi 3 Model B  SPIModule=uint32(0)  Mode=Master  BusSpeed=1000000  Pin=SPI0_CE1  FirstBitToTransfer=Most significant bit (MSB)  ClockMode=0  BlockFunction=Transfer  RegisterAddress=0  OutputDataType=int8  OutputDataLength=1
      settings: SourceProductName=Simulink Support Package for Raspberry Pi Hardware  SourceProductBaseCode=RASPPI
  SPI_MSG_SET_ SENSOR_TYPE : Constant  Value=12  OutMin=[1]  OutMax=[28]  OutDataTypeStr=uint8
  Selector1 : Selector  InputPortWidth=4  IndexOptions=Index vector (dialog)  Indices=[4]  OutputSizes=1
  Sensor type offset : Constant  Value=14  OutDataTypeStr=uint8
  Shift Arithmetic : ArithShift  BitShiftNumberSource=Input port  BitShiftNumber=8  BitShiftDirection=Left
      settings: InputPortMap=u0,p1
  Subtract : Sum  Inputs=+-
  Sum : Sum
  Error : Outport  InitialOutput=[1]
  wires:
  Sensor type offset/1 -> Sum/2
  SensorType/1 -> Sum/1
  Sum/1 -> Mux1/4
  Shift Arithmetic/1 -> Mux1/3
  Constant2/1 -> Shift Arithmetic/1
  SensorPort/1 -> Subtract/1
  Constant3/1 -> Subtract/2
  Subtract/1 -> Shift Arithmetic/2
  NAND/1 -> Error/1
  0xA5/1 -> NAND/2
  Selector1/1 -> NAND/1
  SPI_MSG_SET_ SENSOR_TYPE/1 -> Mux1/2
  Address/1 -> Mux1/1
  SPI Master Transfer1/1 -> Selector1/1
  Mux1/1 -> SPI Master Transfer1/1
